simulink model "gateway"
settings: Solver=ode45  StartTime=0.0  StopTime=2  RelTol=1e-3
libraries: truetime x8, simulink_extras x1
settings Model: Creator=anton  LastModifiedBy=anton
settings DataIOCC: LimitDataPoints=on  SaveFormat=Array  ReturnWorkspaceOutputs=off
settings OptimizationCC: LifeSpan=inf  SimCompilerOptimization=Off
settings DebuggingCC: FcnCallInpInsideContextMsg=Enable All  SFUnexpectedBacktrackingDiag=warning  SFNoUnconditionalDefaultTransitionDiag=warning
settings HardwareCC: ProdBitPerPointer=32  ProdLargestAtomicFloat=None  ProdIntDivRoundTo=Undefined  ProdEndianess=Unspecified  ProdWordSize=32  ProdHWDeviceType=32-bit Generic
settings ModelReferenceCC: PropagateSignalLabelsOutOfModel=off
settings SFSimCC: SimUseLocalCustomCode=off
settings RTWCC: RTWUseLocalCustomCode=off  RTWCompilerOptimization=Off
settings GRTTargetCC: CodeReplacementLibrary=C89/C90 (ANSI)  GeneratePreprocessorConditionals=Disable all  CPPClassGenCompliant=off

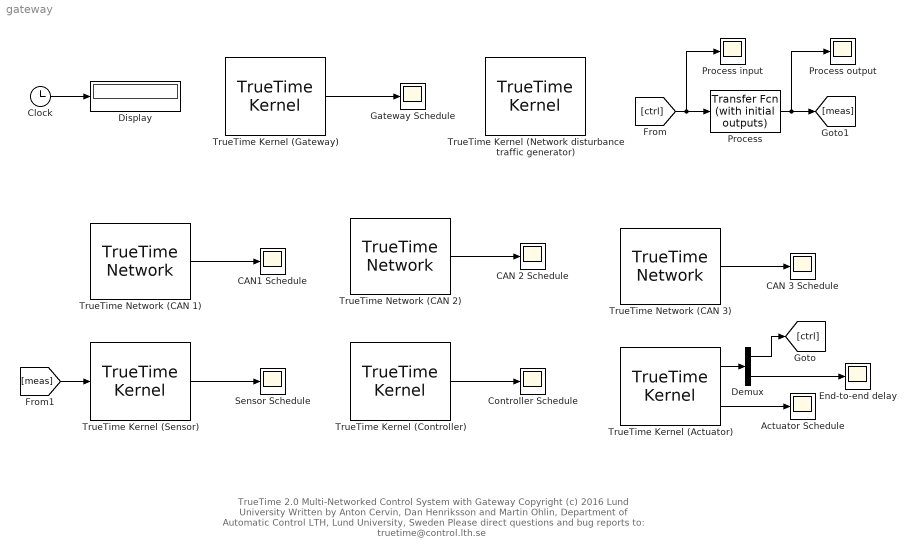
== system gateway ==
  note: TrueTime 2.0  Multi-Networked Control System with Gateway
      | Copyright (c) 2016 Lund University
      | Written by Anton Cervin, Dan Henriksson and Martin Ohlin,
      | Department of Automatic Control LTH, Lund University, Sweden
      | Please direct questions and bug reports to:  truetime@control.lth.se
  Actuator Schedule : Scope
      settings: TimeRange=2  YMin=0.9  YMax=1.1  SaveName=nschedule6
  CAN 2 Schedule : Scope
      settings: TimeRange=2  YMin=1  YMax=3.5  SaveName=nschedule3
  CAN 3 Schedule : Scope
      settings: TimeRange=2  YMin=1  YMax=3.5  SaveName=nschedule5
  CAN1 Schedule : Scope
      settings: TimeRange=2  YMin=1  YMax=3.5  SaveName=nschedule
  Clock : Clock
  Controller Schedule : Scope
      settings: TimeRange=2  YMin=1  YMax=1.5  SaveName=nschedule2
  Demux : Demux  Outputs=2
  Display : Display
  End-to-end delay : Scope
      settings: TimeRange=2  YMin=0  YMax=0.04  SaveName=nschedule9
  Gateway Schedule : Scope
      settings: TimeRange=2  YMin=1  YMax=1.5  SaveName=nschedule4
  Process : simulink_extras/Additional Linear/Transfer Fcn (with initial outputs)  N=[10]  D="[10  1]"  Y0=1  U0=0
  Process input : Scope
      settings: TimeRange=2  YMin=-1.00000  YMax=1.00000  SaveName=nschedule8
  Process output : Scope
      settings: TimeRange=2  YMin=0  YMax=1  SaveName=nschedule7
  Sensor Schedule : Scope
      settings: TimeRange=2  YMin=1  YMax=1.5  SaveName=nschedule1
  TrueTime Kernel (Actuator) : truetime/TrueTime Kernel  Priority=1  sfun=actuator_init  args=[]  ninputsoutputs=[0 2]  ntriggers=0  trigtype=rising  nwnodenbr=[3 1]  clockoffsetdrift=[0 0]  schedoutput=on  battery=off  poweroutput=off  label=3: 1
  TrueTime Kernel (Controller) : truetime/TrueTime Kernel  Priority=1  sfun=controller_init  args=[]  ninputsoutputs=[0 0]  ntriggers=0  trigtype=rising  nwnodenbr=[2 1]  clockoffsetdrift=[0 0]  schedoutput=on  battery=off  poweroutput=off  label=2: 1
  TrueTime Kernel (Gateway) : truetime/TrueTime Kernel  Priority=1  sfun=gateway_init  args=[]  ninputsoutputs=[0 0]  ntriggers=0  trigtype=rising  nwnodenbr=[1 2; 2 2; 3 2]  clockoffsetdrift=[0 0]  schedoutput=on  battery=off  poweroutput=off  label=1: 2\n2: 2\n3: 2
  TrueTime Kernel (Network disturbance traffic generator) : truetime/TrueTime Kernel  Priority=1  sfun=disturbance_init  args=[]  ninputsoutputs=[0 0]  ntriggers=0  trigtype=rising  nwnodenbr=[1 3; 2 3; 3 3]  clockoffsetdrift=[0 0]  schedoutput=off  battery=off  poweroutput=off  label=1: 3\n2: 3\n3: 3
  TrueTime Kernel (Sensor) : truetime/TrueTime Kernel  Priority=1  sfun=sensor_init  args=[]  ninputsoutputs=[1 0]  ntriggers=0  trigtype=rising  nwnodenbr=[1 1]  clockoffsetdrift=[0 0]  schedoutput=on  battery=off  poweroutput=off  label=1: 1
  TrueTime Network (CAN 1) : truetime/TrueTime Network  Priority=1  nwtype=CSMA/AMP (CAN)  nwnbr=1  nnodes=3  rate=125000  minsize=29  lossprob=0  seed=0  bandwidths=[0.5 0.25 0.25]  slotsize=80  schedule=[1 2 1 3]  memsize=80000  buftype=Common buffer  overflow=Retransmit  dynSchedule=[]  miniSlotSize=40  NIT=0  QSortMode=FIFO  sync=0  irtSchedule=0  nrtLength=0  nodeGraph=0  scheduleoutput=on
  TrueTime Network (CAN 2) : truetime/TrueTime Network  Priority=1  nwtype=CSMA/AMP (CAN)  nwnbr=2  nnodes=3  rate=125000  minsize=29  lossprob=0  seed=0  bandwidths=[0.5 0.25 0.25]  slotsize=80  schedule=[1 2 1 3]  memsize=80000  buftype=Common buffer  overflow=Retransmit  dynSchedule=[]  miniSlotSize=40  NIT=0  QSortMode=FIFO  sync=0  irtSchedule=0  nrtLength=0  nodeGraph=0  scheduleoutput=on
  TrueTime Network (CAN 3) : truetime/TrueTime Network  Priority=1  nwtype=CSMA/AMP (CAN)  nwnbr=3  nnodes=3  rate=125000  minsize=29  lossprob=0  seed=0  bandwidths=[0.5 0.25 0.25]  slotsize=80  schedule=[1 2 1 3]  memsize=80000  buftype=Common buffer  overflow=Retransmit  dynSchedule=[]  miniSlotSize=40  NIT=0  QSortMode=FIFO  sync=0  irtSchedule=0  nrtLength=0  nodeGraph=0  scheduleoutput=on
  wires:
  TrueTime Network (CAN 1)/1 -> CAN1 Schedule/1
  Clock/1 -> Display/1
  TrueTime Kernel (Sensor)/1 -> Sensor Schedule/1
  TrueTime Kernel (Controller)/1 -> Controller Schedule/1
  TrueTime Network (CAN 2)/1 -> CAN 2 Schedule/1
  TrueTime Kernel (Gateway)/1 -> Gateway Schedule/1
  TrueTime Network (CAN 3)/1 -> CAN 3 Schedule/1
  TrueTime Kernel (Actuator)/2 -> Actuator Schedule/1
  [meas] -> TrueTime Kernel (Sensor)/1
  Process/1 -> [meas], Process output/1
  [ctrl] -> Process input/1, Process/1
  TrueTime Kernel (Actuator)/1 -> Demux/1
  Demux/1 -> [ctrl]
  Demux/2 -> End-to-end delay/1
